simulink model "ee_motor_pmsm_drive"  (R2020b)
settings: Solver=ode23t  StartTime=0.0  StopTime=tsim  MaxStep=1e-6  RelTol=1e-4  AbsTol=1e-3  EnableMultiTasking=on
PreLoadFcn:
  | tsim = 0.05;
PostLoadFcn:
  | % Create the PMSM data
  | ee_motor_pmsm_drive_params
  | 
  | % Test harness test point
  | rpm0 = 1400;
  | torque0 = 200;
InitFcn:
  | % Set simulation time for 5 full AC cycles
  | tsim = 5*60/rpm0/N;
StopFcn:
  | ee_addSimlogTimeStamp(bdroot)
undefined symbols (not defined in the file): Imax, Ld, Lq, N, PM, Rs, Tmax, Ts, Tsc
libraries: ee_lib x22, fl_lib x12, nesl_utility x12, pid_lib x3, eeTransforms x2, eePwmGeneratorTwoLevel x1
(part 1 of 2)
CloseFcn:
  | try,close(h1_ee_motor_pmsm_drive),end
  | clear h1_ee_motor_pmsm_drive
  | try,close(h2_ee_motor_pmsm_drive),end
  | clear h2_ee_motor_pmsm_drive
  | try,close(h3_ee_motor_pmsm_drive),end
  | clear h3_ee_motor_pmsm_drive
  | try,close(h4_ee_motor_pmsm_drive),end
  | clear h4_ee_motor_pmsm_drive
  | 
  | 
  | clear simlog_ee_motor_pmsm_drive
  | clear logsout_ee_motor_pmsm_drive
  | clear Imax L0 Ld Lq N PM Pmax Rs Tmax TorqueMatrix Ts Tsc dfluxAdiaMatrix dfluxAdibMatrix dfluxAdicMatrix dfluxAdxMatrix efficiency fc fnom fsw iDC idVec iqVec omegam_nom powerDC powerLosses rpm0 rpm_nom t tMax tMin tabulatedLosses time torque0 totalLosses tout tsim vDC xVec
Description:
  | HEV PMSM Drive Test Harness
settings Model: Creator=The MathWorks, Inc.  LastModifiedBy=ge62gas
settings SolverCC: AutoScaleAbsTol=off  MaxConsecutiveMinStep=2
settings DataIOCC: LimitDataPoints=on  MaxDataPoints=35000  SaveFormat=StructureWithTime  SaveOutput=off  DSMLogging=off  ReturnWorkspaceOutputs=off  SignalLoggingName=logsout_ee_motor_pmsm_drive
settings OptimizationCC: LifeSpan=inf
settings DebuggingCC: UnderspecifiedInitializationDetection=Classic  MergeDetectMultiDrivingBlocksExec=none  AllowSymbolicDim=off  PregeneratedLibrarySubsystemCodeDiagnostic=none  SFUnexpectedBacktrackingDiag=warning  SFNoUnconditionalDefaultTransitionDiag=warning  SFExecutionAtInitializationDiag=none  ArithmeticOperatorsInVariantConditions=warning
settings HardwareCC: ProdBitPerPointer=32  ProdBitPerSizeT=32  ProdBitPerPtrDiffT=32  ProdLargestAtomicFloat=None  ProdIntDivRoundTo=Undefined  ProdEndianess=Unspecified  ProdWordSize=32  ProdHWDeviceType=32-bit Generic
settings ModelReferenceCC: PropagateSignalLabelsOutOfModel=off
settings SFSimCC: SimUseLocalCustomCode=off
settings RTWCC: RTWUseLocalCustomCode=off
settings CodeAppCC: StateflowObjectComments=on
settings GRTTargetCC: TargetLangStandard=C89/C90 (ANSI)
settings ConfigComp: CovMetricSettings=dw  CovSaveCumulativeToWorkspaceVar=on  CovSaveSingleToWorkspaceVar=on  CovExternalEMLEnable=off  CovSFcnEnable=off
settings SimscapeCC: SimscapeLogType=all  SimscapeLogSimulationStatistics=on  SimscapeLogName=simlog_ee_motor_pmsm_drive  SimscapeLogDecimation=10  SimscapeLogDataHistory=1000000

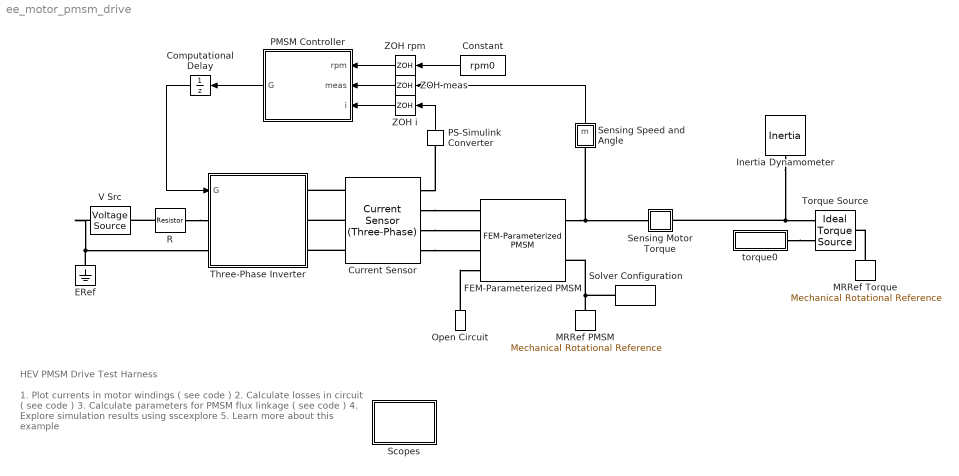
== system ee_motor_pmsm_drive ==
  note: HEV PMSM Drive Test Harness
  note: 1. Plot currents in motor windings ( see code )
      | 2. Calculate losses in circuit ( see code )
      | 3. Calculate parameters for PMSM flux linkage ( see code )
      | 4. Explore simulation results using sscexplore
      | 5. Learn more about this example
  Computational Delay : UnitDelay  SampleTime=Ts  HasFrameUpgradeWarning=on
  Constant : Constant  Value=rpm0
  Current Sensor : ee_lib/Sensors & Transducers/Current Sensor (Three-Phase)
      settings: SourceProductName=Electrical  InternalSimscapePortConfiguration="{\"Bottom\":[],\"Left\":[{\"id\":\"a1\",\"label\":\"a1\",\"type\":\"foundation.electrical.electrical\"},{\"id\":\"b1\",\"label\":\"b1\",\"type\":\"foundation.electrical.electrical\"},{\"id\":\"c1\",\"label\":\"c1\",\"type\":\"foundation.electrical.electrical\"}],\"Right\":[{\"id\":\"I_output\",\"label\":\"I\",\"type\":\"output\"},{\"id\":\"a2\",\"label\":\"a2\",\"type\":\"foundation.electrical.electrical\"},{\"id\":\"b2\",\"label\":\"b2\",\"type\":\"foundation.electrical.electrical\"},{\"id\":\"c2\",\"label\":\"c2\",\"type\":\"foundation.electrical.electrical\"}],\"Top\":[]}"
  ERef : fl_lib/Electrical/Electrical Elements/Electrical Reference
      settings: SourceProductName=Foundation Library
  FEM-Parameterized PMSM : ee_lib/Electromechanical/Permanent Magnet/FEM-Parameterized PMSM  parameterization=1  winding_type=ee.enum.statorconnection.wye  iVec=[-2, 0, 2] A  xVec=xVec rad  dfluxdiMatrix=0.0002 * ones(3, 4) Wb/A  dfluxdxMatrix=[0, -.16, .16, 0; 0, -.16, .16, 0; 0, -.16, .16, 0] Wb/rad  calculate_torque_matrix=1  TorqueMatrix=zeros(3, 3, 3, 4) N*m  idVec1=[-200, 0, 200] A  iqVec1=[-200, 0, 200] A  LdMatrix=0.0002 * ones(3, 3) H  LqMatrix=0.0002 * ones(3, 3) H  PmMatrix=0.1 * ones(3, 3) Wb  N=6  interp_method=simscape.enum.interpolation.smooth  Rs=Rs Ohm  Ms=0.00002 H  L0=0.00016 H  losses_oc=[500 1500 0] W  losses_sc=[200 600 0] W  f_losses=140 Hz  Isc_losses=350 A  Inertia=0.01 kg*m^2  lam=0 N*m/(rad/s)  i_d_specify=on  i_d_priority=High  i_d=0 A  i_d_nominal_specify=off  i_d_nominal_unit=A  i_d_nominal_value=1  i_q_specify=on  i_q_priority=High  i_q=0 A  i_q_nominal_specify=off  i_q_nominal_unit=A  i_q_nominal_value=1  torque_specify=off  torque_priority=None  torque=0 N*m  torque_nominal_specify=off  torque_nominal_unit=N*m  torque_nominal_value=1  angular_velocity_specify=on  angular_velocity_priority=High  angular_velocity=rpm0 rpm  angular_velocity_nominal_specify=off  angular_velocity_nominal_unit=rpm  angular_velocity_nominal_value=1  angular_position_specify=on  angular_position_priority=High  angular_position=-pi/2/N rad  angular_position_nominal_specify=off  angular_position_nominal_unit=deg  angular_position_nominal_value=1  Tmeas=298.15 K  alpha=3.93e-3 1/K  alpha_flux=-0.001 1/K  stator_thermal_mass=100 J/K  stator_initial_temperatures=[298.15, 298.15, 298.15] K  rotor_thermal_mass=200 J/K  rotor_initial_temperature=298.15 K  Rm_percent_rotor=90  Rd_percent_rotor=30  idVec=idVec A  iqVec=iqVec A  dfluxAdiaMatrix3D=dfluxAdiaMatrix Wb/A  dfluxAdibMatrix3D=dfluxAdibMatrix Wb/A  dfluxAdicMatrix3D=dfluxAdicMatrix Wb/A  dfluxAdxMatrix3D=dfluxAdxMatrix Wb/rad  TorqueMatrix3D=TorqueMatrix N*m  iaVec=[-200, 0, 200] A  ibVec=[-200, 0, 200] A  icVec=[-200, 0, 200] A  dfluxAdiaMatrix=zeros(3, 3, 3, 4) Wb/A  dfluxAdibMatrix=zeros(3, 3, 3, 4) Wb/A  dfluxAdicMatrix=zeros(3, 3, 3, 4) Wb/A  dfluxAdxMatrix=zeros(3, 3, 3, 4) Wb/rad  param_dq0=1  winding_type_dq0=1  nPolePairs=4  parks_type=1  idVec2=[-200, 0, 200] A  iqVec2=[-200, 0, 200] A  magVec2=[0, 100, 200] A  betaVec2=[-180, -90, 0, 90, 180] deg  xVec2=[0, 5, 10, 15, 20, 25, 30] deg  fluxD_dq0=zeros(3, 3, 7) Wb  fluxQ_dq0=zeros(3, 3, 7) Wb  fluxA_dq0=zeros(3, 3, 7) Wb  Torque_dq0=zeros(3, 3, 7) N*m  fluxD_IBX=zeros(3, 5, 7) Wb  fluxQ_IBX=zeros(3, 5, 7) Wb  fluxA_IBX=zeros(3, 5, 7) Wb  Torque_IBX=zeros(3, 5, 7) N*m
      settings: SourceProductName=Electrical  LogSimulationData=on  InternalSimscapePortConfiguration="{\"Bottom\":[],\"Left\":[{\"id\":\"a\",\"label\":\"a\",\"type\":\"foundation.electrical.electrical\"},{\"id\":\"b\",\"label\":\"b\",\"type\":\"foundation.electrical.electrical\"},{\"id\":\"c\",\"label\":\"c\",\"type\":\"foundation.electrical.electrical\"},{\"id\":\"n\",\"label\":\"n\",\"type\":\"foundation.electrical.electrical\"}],\"Right\":[{\"id\":\"R\",\"label\":\"R\",\"type\":\"foundation.mechanical.rotational.rotational\"},{\"id\":\"C\",\"label\":\"C\",\"type\":\"foundation.mechanical.rotational.rotational\"}],\"Top\":[]}"
  Inertia Dynamometer : fl_lib/Mechanical/Rotational Elements/Inertia  inertia=1 kg*m^2  num_ports=foundation.enum.numPorts2.one  w_specify=on  w_priority=High  w=rpm0 rpm  w_nominal_specify=off  w_nominal_unit=rad/s  w_nominal_value=1  t_specify=off  t_priority=High  t=0 N*m  t_nominal_specify=off  t_nominal_unit=N*m  t_nominal_value=1
      settings: SourceProductName=Foundation Library
  MRRef PMSM : fl_lib/Mechanical/Rotational Elements/Mechanical Rotational Reference
      settings: SourceProductName=Foundation Library
  MRRef Torque : fl_lib/Mechanical/Rotational Elements/Mechanical Rotational Reference
      settings: SourceProductName=Foundation Library
  Open Circuit : fl_lib/Electrical/Electrical Elements/Open Circuit  v_specify=off  v_priority=None  v=0 V  v_nominal_specify=off  v_nominal_unit=V  v_nominal_value=1
      settings: SourceProductName=Foundation Library
  PMSM Controller : Subsystem
  PS-Simulink Converter : nesl_utility/PS-Simulink Converter  PhysicalDomain=network_engine_domain  SubClassName=ps_output  LeftPortType=input  RightPortType=output  PseudoPeriodic=off  Frequencies=[]  Unit=A  AffineConversion=off
      settings: SourceProductName=Utilities
  R : fl_lib/Electrical/Electrical Elements/Resistor  R=0.01 Ohm  i_specify=off  i_priority=None  i=0 A  i_nominal_specify=off  i_nominal_unit=A  i_nominal_value=1  v_specify=off  v_priority=None  v=0 V  v_nominal_specify=off  v_nominal_unit=V  v_nominal_value=1
      settings: SourceProductName=Foundation Library
  Scopes : Subsystem
  Sensing Motor Torque : Subsystem
      mask Display: disp('trq');
  Sensing Speed and Angle : Subsystem
      mask Display: disp('m')
  Solver Configuration : nesl_utility/Solver Configuration  PhysicalDomain=network_engine_domain  SubClassName=solver  LeftPortType=input  RightPortType=generic  Tones=[]  Harmonics=[]  SimulateNoise=off  Profile=off  UseLocalSampling=off  EnableSwitchedLinearOptims=on  FrequencyDomain=off  UseCCode=off  RelTol=0.001  AbsTol=1e-06  MinStep=1e-09  ToWorkspace=off  RevertToSquareIcSolve=off  NumHomotopyIterations=100  PhasorMode=off  PhasorModeNumHarmonics=1  DoDC=off  ResidualTolerance=1e-9  UseLocalSolver=off  LocalSolverChoice=NE_BACKWARD_EULER_ADVANCER  LocalSolverSampleTime=Ts/1000  DoFixedCost=on  MaxNonlinIter=4  MaxModeIter=2  ComputeImpulses=off  ImpulseIterations=2  LinearAlgebra=auto  EquationFormulation=NE_TIME_EF  DelaysMemoryBudget=1024  AutomaticFiltering=on  FilteringTimeConstant=0.001  PartitionStorageMethod=AS_NEEDED  PartitionMemoryBudget=1024  PartitionMethod=FAST
      settings: SourceProductName=Utilities
  Three-Phase Inverter : Subsystem  Tag=PublishSubsystem
  Torque Source : fl_lib/Mechanical/Mechanical Sources/Ideal Torque Source
      settings: SourceProductName=Foundation Library
  V Src : ee_lib/Sources/Voltage Source  dc_voltage=500 V  ac_voltage=0 V  ac_shift=0 deg  ac_frequency=0 Hz  noise_mode=0  PSD=0 V^2/Hz  repeatability=1  auto_seed=529650792  user_seed=0  sample_time=0.001 s  i_specify=off  i_priority=None  i=0 A  i_nominal_specify=off  i_nominal_unit=A  i_nominal_value=1  v_specify=off  v_priority=None  v=0 V  v_nominal_specify=off  v_nominal_unit=V  v_nominal_value=1
      settings: AttributesFormatString=%<dc_voltage> %<dc_voltage_unit>  SourceProductName=Electrical
  ZOH i : ZeroOrderHold  SampleTime=Tsc
  ZOH meas : ZeroOrderHold  SampleTime=Tsc
  ZOH rpm : ZeroOrderHold  SampleTime=Tsc
  torque0 : Subsystem
      mask Display: disp('torque0');
  wires:
  PMSM Controller/1(G) -> Computational Delay/1
  ZOH i/1 -> PMSM Controller/3(i)
  Computational Delay/1 -> Three-Phase Inverter/1(G)
  ZOH meas/1 -> PMSM Controller/2(meas)
  ZOH rpm/1 -> PMSM Controller/1(rpm)
  Sensing Speed and Angle/1(m) -> ZOH meas/1
  Constant/1 -> ZOH rpm/1
  PS-Simulink Converter/1 -> ZOH i/1
  connections:
  FEM-Parameterized PMSM/RConn1 -- Sensing Speed and Angle/LConn1 -- Sensing Motor Torque/LConn1
  V Src/RConn1 -- Three-Phase Inverter/LConn2 -- ERef/LConn1
  Current Sensor/LConn1 -- Three-Phase Inverter/RConn1
  Current Sensor/RConn2 -- FEM-Parameterized PMSM/LConn1
  Current Sensor/LConn2 -- Three-Phase Inverter/RConn2
  Current Sensor/RConn3 -- FEM-Parameterized PMSM/LConn2
  Current Sensor/LConn3 -- Three-Phase Inverter/RConn3
  Current Sensor/RConn4 -- FEM-Parameterized PMSM/LConn3
  Inertia Dynamometer/LConn1 -- Sensing Motor Torque/RConn1 -- Torque Source/RConn2
  R/LConn1 -- V Src/LConn1
  R/RConn1 -- Three-Phase Inverter/LConn1
  MRRef PMSM/LConn1 -- Solver Configuration/RConn1 -- FEM-Parameterized PMSM/RConn2
  Open Circuit/LConn1 -- FEM-Parameterized PMSM/LConn4
  MRRef Torque/LConn1 -- Torque Source/LConn1
  torque0/RConn1 -- Torque Source/RConn1
  Current Sensor/RConn1 -- PS-Simulink Converter/LConn1

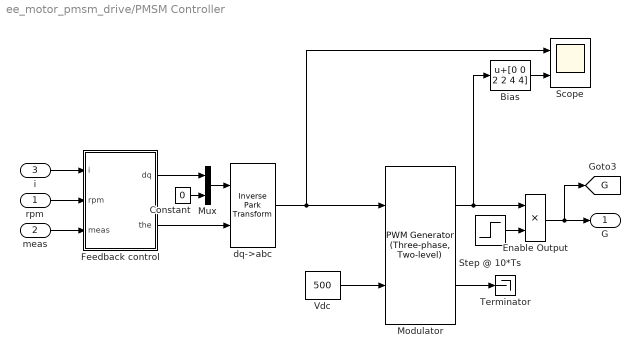
== system ee_motor_pmsm_drive/PMSM Controller ==
  rpm : Inport
  meas : Inport  Port=2
  i : Inport  Port=3
  Bias : Bias  Bias=[0 0 2 2 4 4]
  Constant : Constant  Value=0  SampleTime=-1
  Enable Output : Product
  Feedback control : Subsystem
  Modulator : eePwmGeneratorTwoLevel/PWM Generator (Three-phase, Two-level)  PWMMode=Continuous PWM (CPWM)  CPWMMode=SPWM: sinusoidal PWM  DPWMMode=60 DPWM: 60 degree discontinuous PWM  fsw=fsw  Ts=Ts
      settings: SourceProductBaseCode=PS
  Mux : Mux  Inputs=2
  Scope : Scope  NumInputPorts=2
  Step @ 10*Ts : Step  Time=10*Ts  SampleTime=Ts
  Terminator : Terminator
  Vdc : Constant  Value=500  SampleTime=Tsc
  dq->abc : eeTransforms/Inverse Park Transform  AxisAlignment=Q-axis  PowerInvariant=off
  G : Outport  VectorParamsAs1DForOutWhenUnconnected=off
  tag scope: G=global
  wires:
  dq->abc/1 -> Scope/1, Modulator/1
  Vdc/1 -> Modulator/2
  Step @ 10*Ts/1 -> Enable Output/2
  Modulator/2 -> Terminator/1
  i/1 -> Feedback control/1(i)
  rpm/1 -> Feedback control/2(rpm)
  meas/1 -> Feedback control/3(meas)
  Feedback control/2(the) -> dq->abc/2
  Modulator/1 -> Bias/1, Enable Output/1
  Enable Output/1 -> [G], G/1
  Constant/1 -> Mux/2
  Mux/1 -> dq->abc/1
  Feedback control/1(dq) -> Mux/1
  Bias/1 -> Scope/2

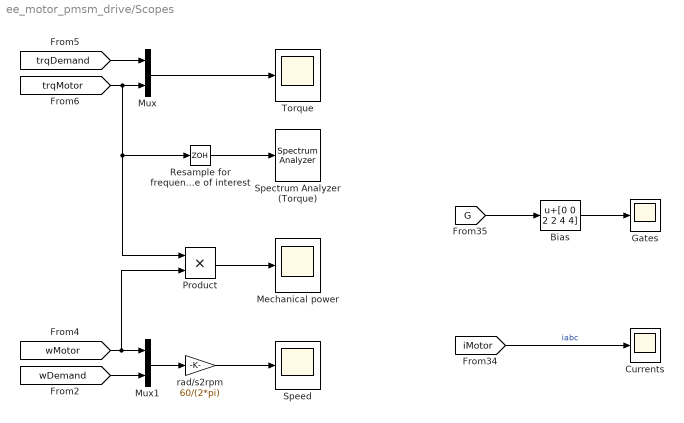
== system ee_motor_pmsm_drive/Scopes ==
  Bias : Bias  Bias=[0 0 2 2 4 4]
  Currents : Scope
  Gates : Scope
  Mechanical power : Scope
  Mux : Mux  Inputs=2
  Mux1 : Mux  Inputs=2
  Product : Product
  Resample for frequency range of interest : ZeroOrderHold  SampleTime=2.5e-5
  Spectrum Analyzer (Torque) : SpectrumAnalyzer  Tag=PublishScope
  Speed : Scope
  Torque : Scope
  rad/s2rpm : Gain  Gain=60/(2*pi)
  wires:
  rad/s2rpm/1 -> Speed/1
  Mux/1 -> Torque/1
  [iMotor] -> Currents/1  "iabc"
  [trqDemand] -> Mux/1
  Mux1/1 -> rad/s2rpm/1
  [wMotor] -> Mux1/1, Product/2
  [G] -> Bias/1
  Bias/1 -> Gates/1
  Product/1 -> Mechanical power/1
  Resample for frequency range of interest/1 -> Spectrum Analyzer (Torque)/1
  [wDemand] -> Mux1/2
  [trqMotor] -> Product/1, Resample for frequency range of interest/1, Mux/2

== system ee_motor_pmsm_drive/Sensing Motor Torque ==
  Ideal Torque Sensor : fl_lib/Mechanical/Mechanical Sensors/Ideal Torque Sensor
      settings: SourceProductName=Foundation Library
  PS-Simulink Converter2 : nesl_utility/PS-Simulink Converter  PhysicalDomain=network_engine_domain  SubClassName=ps_output  LeftPortType=input  RightPortType=output  PseudoPeriodic=off  Frequencies=[]  Unit=N*m  AffineConversion=off
      settings: SourceProductName=Utilities
  R : PMIOPort  Side=Left
  C : PMIOPort  Port=2  Side=Right
  tag scope: trqMotor=global
  wires:
  PS-Simulink Converter2/1 -> [trqMotor]
  connections:
  Ideal Torque Sensor/RConn2 -- PS-Simulink Converter2/LConn1
  R/RConn1 -- Ideal Torque Sensor/LConn1
  Ideal Torque Sensor/RConn1 -- C/RConn1

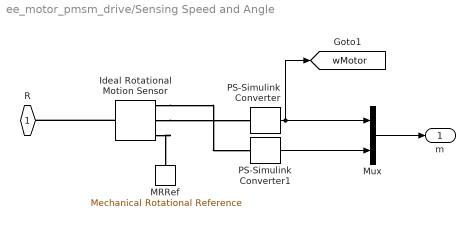
== system ee_motor_pmsm_drive/Sensing Speed and Angle ==
  Ideal Rotational Motion Sensor : fl_lib/Mechanical/Mechanical Sensors/Ideal Rotational Motion Sensor  wrap_angle=simscape.enum.onoff.off  offset=0 deg
      settings: SourceProductName=Foundation Library
  MRRef : fl_lib/Mechanical/Rotational Elements/Mechanical Rotational Reference
      settings: SourceProductName=Foundation Library
  Mux : Mux  Inputs=2
  PS-Simulink Converter : nesl_utility/PS-Simulink Converter  PhysicalDomain=network_engine_domain  SubClassName=ps_output  LeftPortType=input  RightPortType=output  PseudoPeriodic=off  Frequencies=[]  Unit=rad/s  AffineConversion=off
      settings: SourceProductName=Utilities
  PS-Simulink Converter1 : nesl_utility/PS-Simulink Converter  PhysicalDomain=network_engine_domain  SubClassName=ps_output  LeftPortType=input  RightPortType=output  PseudoPeriodic=off  Frequencies=[]  Unit=rad  AffineConversion=off
      settings: SourceProductName=Utilities
  R : PMIOPort  Side=Left
  m : Outport  VectorParamsAs1DForOutWhenUnconnected=off
  tag scope: wMotor=global
  wires:
  Mux/1 -> m/1
  PS-Simulink Converter/1 -> Mux/1, [wMotor]
  PS-Simulink Converter1/1 -> Mux/2
  connections:
  Ideal Rotational Motion Sensor/RConn3 -- PS-Simulink Converter1/LConn1
  Ideal Rotational Motion Sensor/RConn1 -- MRRef/LConn1
  Ideal Rotational Motion Sensor/RConn2 -- PS-Simulink Converter/LConn1
  Ideal Rotational Motion Sensor/LConn1 -- R/RConn1

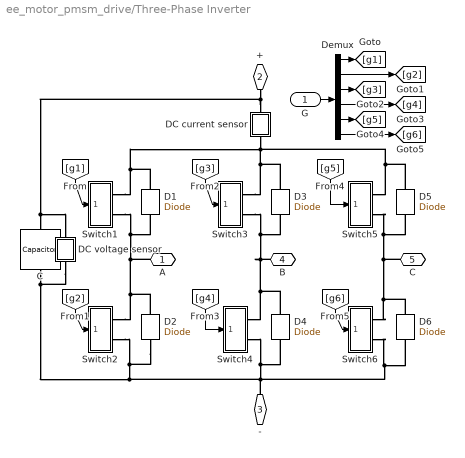
== system ee_motor_pmsm_drive/Three-Phase Inverter ==
  G : Inport
  " C" : ee_lib/Passive/Capacitor  cap_option=0  c=10 F  Cvec=[ 1e-5 1e-6 ] F  Vvec=[ 0 10 ] V  CV_table_symmetry=1  f_vec=[1, 10] kHz  DFext_vec=[.8, 1.2]  C_tol=5  enable_C_tol=0  tol_distribution=1  nSigma=4  r=0.001 Ohm  g=0 1/Ohm  averaging_period=0 s  enable_operating_limits=0  operating_limit_action=2  max_working_voltage_range=[ -25 25 ] V  power_rating=1 W  enable_faults=0  fault_action=1  Cscale_faulted=100  R_faulted=0.001 Ohm  G_faulted=0 1/Ohm  tau_fault=0.001 s  enable_temporal_fault=0  t_fault=1 s  enable_behavioral_fault=0  max_permissible_voltage_range=[ -100 100 ] V  t_fail_on_voltage=1 s  i_specify=off  i_priority=Low  i=0 A  i_nominal_specify=off  i_nominal_unit=A  i_nominal_value=1  v_specify=off  v_priority=None  v=0 V  v_nominal_specify=off  v_nominal_unit=V  v_nominal_value=1  vc_specify=on  vc_priority=High  vc=500 V  vc_nominal_specify=off  vc_nominal_unit=V  vc_nominal_value=1
      settings: SourceProductName=Electrical
  D{1..6} (6 alike) : ee_lib/Semiconductors & Converters/Diode  ModelType=ee.enum.diode.modelType.exponential  IfMat=[.07, .12, .19, 1.75, 4.24, 7.32, 11.2; .16, .3, .72, 2.14, 4.02, 6.35, 9.12] A  TjVec=[25, 125] degC  VfVec=[.5, .7, .9, 1.3, 1.7, 2.1, 2.5] V  Vf=0.6 V  Ron=0.3 Ohm  Goff=1e-8 S  prmExp=2  I12=[ 0.0137 0.545 ] A  V12=[ 0.6 0.7 ] V  IS=1e-7 A  ec=1  I1=0.0137 A  V1=0.6 V  RS=0.001 Ohm  Tmeas=25 degC  N_series=1  N_parallel=1  Rz=0.3 Ohm  BV=Inf V  C_param=1  CJ=50 pF  CJ0=50 pF  VJ=1 V  Mgrad=0.5  Vvec=[ 0.1 10 100 ] V  Cvec=[ 3.5 1 0.4 ] pF  FC=0.5  Q_param=ee.enum.diode.recoveryParam.off  iRM=-7.15 A  iF=4 A  didt=-750 A/us  trr_factor=3  trr=115 ns  Qrr=1500 s*uA  TT=50 ns  tau=100 ns  T_param=1  IS_T2=1.25e-7 A  I1_T2=0.245 A  V1_T2=0.5 V  Tmeas2=125 degC  EG_param=1  EG=1.11 eV  XTI_param=1  XTI=3  dBVdT=0 V/K  Tdevice=25 degC  i_specify=off  i_priority=None  i=0 A  i_nominal_specify=off  i_nominal_unit=A  i_nominal_value=1  v_specify=off  v_priority=None  v=0 V  v_nominal_specify=off  v_nominal_unit=V  v_nominal_value=1  i_capacitor_specify=off  i_capacitor_priority=High  i_capacitor=0 A  i_capacitor_nominal_specify=off  i_capacitor_nominal_unit=A  i_capacitor_nominal_value=1  v_capacitor_specify=off  v_capacitor_priority=None  v_capacitor=0 V  v_capacitor_nominal_specify=off  v_capacitor_nominal_unit=V  v_capacitor_nominal_value=1  power_dissipated_specify=off  power_dissipated_priority=None  power_dissipated=0 W  power_dissipated_nominal_specify=off  power_dissipated_nominal_unit=W  power_dissipated_nominal_value=1  thermal_network_parameterization=ee.enum.thermalNetworkTopology.cauer  Rth=[0, 10] K/W  Rth_Foster=[4, 6] K/W  thermal_mass_parameterization=ee.enum.thermalNetwork.timeconstant  thermal_mass=[0, 1] J/K  thermal_mass_Foster=[1.5, 3] J/K  thermal_time_constant=[0, 10] s  thermal_time_constant_Foster=[6, 18] s  thermal_mass_initial_temperatures=[25, 25] degC
      settings: SourceProductName=Electrical  LogSimulationData=on
  DC current sensor : Subsystem
      mask Display: disp('i');
  DC voltage sensor : Subsystem
      mask Display: disp('v')
  Demux : Demux  Outputs=6
  Switch1 : Subsystem
  Switch2 : Subsystem
  Switch3 : Subsystem
  Switch4 : Subsystem
  Switch5 : Subsystem
  Switch6 : Subsystem
  A : PMIOPort  Tag=PMCPort  Side=Right
  + : PMIOPort  Tag=PMCPort  Port=2  Side=Left
  - : PMIOPort  Tag=PMCPort  Port=3  Side=Left
  B : PMIOPort  Tag=PMCPort  Port=4  Side=Right
  C : PMIOPort  Tag=PMCPort  Port=5  Side=Right
  wires:
  Demux/6 -> [g6]
  Demux/5 -> [g5]
  Demux/4 -> [g4]
  Demux/3 -> [g3]
  Demux/2 -> [g2]
  G/1 -> Demux/1
  Demux/1 -> [g1]
  [g1] -> Switch1/1(g)
  [g2] -> Switch2/1(g)
  [g3] -> Switch3/1(g)
  [g4] -> Switch4/1(g)
  [g5] -> Switch5/1(g)
  [g6] -> Switch6/1(g)
  connections:
  -/RConn1 -- D6/LConn1 -- Switch6/RConn2 -- Switch4/RConn2 -- D4/LConn1 -- DC voltage sensor/LConn1 -- " C"/RConn1 -- D2/LConn1 -- Switch2/RConn2
  A/RConn1 -- Switch1/RConn2 -- D1/LConn1 -- D2/RConn1 -- Switch2/RConn1
  B/RConn1 -- Switch4/RConn1 -- D4/RConn1 -- Switch3/RConn2 -- D3/LConn1
  C/RConn1 -- Switch6/RConn1 -- D6/RConn1 -- Switch5/RConn2 -- D5/LConn1
  +/RConn1 -- DC voltage sensor/RConn1 -- " C"/LConn1 -- DC current sensor/RConn1
  D3/RConn1 -- Switch3/RConn1 -- Switch1/RConn1 -- D1/RConn1 -- DC current sensor/LConn1 -- Switch5/RConn1 -- D5/RConn1

== system ee_motor_pmsm_drive/torque0 ==
  Constant1 : Constant  Value=torque0
  Simulink-PS Converter : nesl_utility/Simulink-PS Converter  PhysicalDomain=network_engine_domain  SubClassName=ps_input  LeftPortType=input  RightPortType=output  PseudoPeriodic=off  Frequencies=[]  NoiseDistribution=none  NoiseParameters=[]  Unit=N*m  AffineConversion=off  FilteringAndDerivatives=zero  SimscapeFilterOrder=1  InputFilterTimeConstant=0.001  UdotUserProvided=1
      settings: SourceProductName=Utilities
  R : PMIOPort  Side=Right
  tag scope: trqDemand=global
  wires:
  Constant1/1 -> Simulink-PS Converter/1, [trqDemand]
  connections:
  Simulink-PS Converter/RConn1 -- R/RConn1

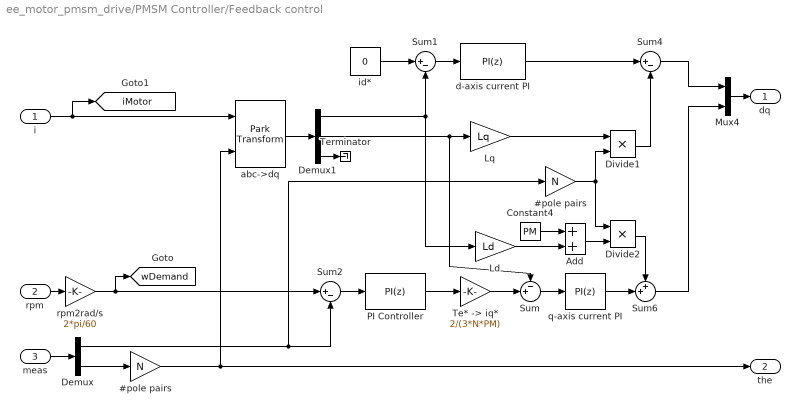
== system ee_motor_pmsm_drive/PMSM Controller/Feedback control ==
  i : Inport
  rpm : Inport  Port=2
  meas : Inport  Port=3
  " #pole pairs " : Gain  Gain=N
  #pole pairs : Gain  Gain=N
  Add : Sum
  Constant4 : Constant  Value=PM  SampleTime=Tsc
  Demux : Demux  Outputs=2
  Demux1 : Demux  Outputs=3
  Divide1 : Product  Inputs=**
  Divide2 : Product  Inputs=**
  Ld : Gain  Gain=Ld
  Lq : Gain  Gain=Lq
  Mux4 : Mux  Inputs=2
  PI Controller : pid_lib/PID Controller  Controller=PI  Form=Parallel  TimeDomain=Discrete-time  UseExternalTs=off  SampleTime=Tsc  IntegratorMethod=Forward Euler  FilterMethod=Forward Euler  ControllerParametersSource=internal  P=120  I=1200  D=0  UseFilter=on  N=100  TunerSelectOption=Transfer Function Based (PID Tuner App)  InitialConditionSource=internal  InitialConditionForIntegrator=torque0  InitialConditionForFilter=0  DifferentiatorICPrevScaledInput=0  ExternalReset=none  TrackingMode=off  Kt=1  LimitOutput=on  SatLimitsSource=internal  UpperSaturationLimit=Tmax*1.5  LowerSaturationLimit=-Tmax*1.5  LinearizeAsGain=on  AntiWindupMode=back-calculation  Kb=1000  POutMin=[]  POutMax=[]  IOutMin=[]  IOutMax=[]  DOutMin=[]  DOutMax=[]  NOutMin=[]  NOutMax=[]  SumOutMin=[]  SumOutMax=[]  SaturationOutMin=[]  SaturationOutMax=[]  PParamMin=[]  PParamMax=[]  IParamMin=[]  IParamMax=[]  DParamMin=[]  DParamMax=[]  NParamMin=[]  NParamMax=[]  KbParamMin=[]  KbParamMax=[]  KtParamMin=[]  KtParamMax=[]  KbOutMin=[]  KbOutMax=[]  KtOutMin=[]  KtOutMax=[]  IntegratorOutMin=[]  IntegratorOutMax=[]  FilterOutMin=[]  FilterOutMax=[]  SumI1OutMin=[]  SumI1OutMax=[]  SumI2OutMin=[]  SumI2OutMax=[]  SumI3OutMin=[]  SumI3OutMax=[]  SumI4OutMin=[]  SumI4OutMax=[]  SumDOutMin=[]  SumDOutMax=[]  DifferentiatorOutMin=[]  DifferentiatorOutMax=[]  FilterDiffOutCoefMin=[]  FilterDiffOutCoefMax=[]  ReciprocalOutMin=[]  ReciprocalOutMax=[]  SumDenOutMin=[]  SumDenOutMax=[]  SumNumOutMin=[]  SumNumOutMax=[]  DivideOutMin=[]  DivideOutMax=[]  UdiffTsProdOutMin=[]  UdiffTsProdOutMax=[]  NTsProdOutMin=[]  NTsProdOutMax=[]  UintegralTsProdOutMin=[]  UintegralTsProdOutMax=[]  UngainTsProdOutMin=[]  UngainTsProdOutMax=[]  IntegratorContinuousStateAttributes=''  IntegratorStateMustResolveToSignalObject=off  IntegratorRTWStateStorageClass=Auto  FilterContinuousStateAttributes=''  FilterStateMustResolveToSignalObject=off  FilterRTWStateStorageClass=Auto  ParallelPVariant=InternalParameters  IdealPVariant=Disabled  IVariant=InternalParameters  DVariant=Disabled  IntegratorVariant=Discrete  SatVariant=Enabled  AWVariant=BackCalculation  PCopyVariant=Disabled  TRVariant=Disabled  FdbkBlocksVariant=Forward  IdealPFdbkVariant=Disabled  SatFdbkVariant=Disabled  DerivativeFilterVariant=Disabled  NVariant=Disabled  NCopyVariant=Disabled_SignalSpec  FilterICVariant=Disabled  IntegratorICVariant=InternalICs  ExternalResetVariant=Disabled  TRSumVariant=Passthrough  SumFdbkVariant=Disabled  SumVariant=Sum_PI  TsampFilterVariant=InternalTs  TsampNgainVariant=Passthrough  TsampIntegralVariant=Passthrough  ExternalSaturationOutDataTypeStr=Inherit: Same as second input
  Sum : Sum  Inputs=-+|
  Sum1 : Sum  Inputs=|+-
  Sum2 : Sum  Inputs=|+-
  Sum4 : Sum  Inputs=|+-
  Sum6 : Sum  Inputs=++|
  "Te* -> iq*" : Gain  Gain=2/(3*N*PM)
  Terminator : Terminator
  abc->dq : eeTransforms/Park Transform  AxisAlignment=Q-axis  PowerInvariant=off
  d-axis current PI : pid_lib/PID Controller  Controller=PI  Form=Parallel  TimeDomain=Discrete-time  UseExternalTs=off  SampleTime=Tsc  IntegratorMethod=Forward Euler  FilterMethod=Forward Euler  ControllerParametersSource=internal  P=0.1  I=10  D=0  UseFilter=on  N=100  TunerSelectOption=Transfer Function Based (PID Tuner App)  InitialConditionSource=internal  InitialConditionForIntegrator=0  InitialConditionForFilter=0  DifferentiatorICPrevScaledInput=0  ExternalReset=none  TrackingMode=off  Kt=1  LimitOutput=on  SatLimitsSource=internal  UpperSaturationLimit=5*Rs*Imax  LowerSaturationLimit=-5*Rs*Imax  LinearizeAsGain=on  AntiWindupMode=back-calculation  Kb=1000  POutMin=[]  POutMax=[]  IOutMin=[]  IOutMax=[]  DOutMin=[]  DOutMax=[]  NOutMin=[]  NOutMax=[]  SumOutMin=[]  SumOutMax=[]  SaturationOutMin=[]  SaturationOutMax=[]  PParamMin=[]  PParamMax=[]  IParamMin=[]  IParamMax=[]  DParamMin=[]  DParamMax=[]  NParamMin=[]  NParamMax=[]  KbParamMin=[]  KbParamMax=[]  KtParamMin=[]  KtParamMax=[]  KbOutMin=[]  KbOutMax=[]  KtOutMin=[]  KtOutMax=[]  IntegratorOutMin=[]  IntegratorOutMax=[]  FilterOutMin=[]  FilterOutMax=[]  SumI1OutMin=[]  SumI1OutMax=[]  SumI2OutMin=[]  SumI2OutMax=[]  SumI3OutMin=[]  SumI3OutMax=[]  SumI4OutMin=[]  SumI4OutMax=[]  SumDOutMin=[]  SumDOutMax=[]  DifferentiatorOutMin=[]  DifferentiatorOutMax=[]  FilterDiffOutCoefMin=[]  FilterDiffOutCoefMax=[]  ReciprocalOutMin=[]  ReciprocalOutMax=[]  SumDenOutMin=[]  SumDenOutMax=[]  SumNumOutMin=[]  SumNumOutMax=[]  DivideOutMin=[]  DivideOutMax=[]  UdiffTsProdOutMin=[]  UdiffTsProdOutMax=[]  NTsProdOutMin=[]  NTsProdOutMax=[]  UintegralTsProdOutMin=[]  UintegralTsProdOutMax=[]  UngainTsProdOutMin=[]  UngainTsProdOutMax=[]  IntegratorContinuousStateAttributes=''  IntegratorStateMustResolveToSignalObject=off  IntegratorRTWStateStorageClass=Auto  FilterContinuousStateAttributes=''  FilterStateMustResolveToSignalObject=off  FilterRTWStateStorageClass=Auto  ParallelPVariant=InternalParameters  IdealPVariant=Disabled  IVariant=InternalParameters  DVariant=Disabled  IntegratorVariant=Discrete  SatVariant=Enabled  AWVariant=BackCalculation  PCopyVariant=Disabled  TRVariant=Disabled  FdbkBlocksVariant=Forward  IdealPFdbkVariant=Disabled  SatFdbkVariant=Disabled  DerivativeFilterVariant=Disabled  NVariant=Disabled  NCopyVariant=Disabled_SignalSpec  FilterICVariant=Disabled  IntegratorICVariant=InternalICs  ExternalResetVariant=Disabled  TRSumVariant=Passthrough  SumFdbkVariant=Disabled  SumVariant=Sum_PI  TsampFilterVariant=InternalTs  TsampNgainVariant=Passthrough  TsampIntegralVariant=Passthrough  ExternalSaturationOutDataTypeStr=Inherit: Same as second input
  id* : Constant  Value=0  SampleTime=Tsc
  q-axis current PI : pid_lib/PID Controller  Controller=PI  Form=Parallel  TimeDomain=Discrete-time  UseExternalTs=off  SampleTime=Tsc  IntegratorMethod=Forward Euler  FilterMethod=Forward Euler  ControllerParametersSource=internal  P=0.1  I=10  D=0.000539029417831173  UseFilter=on  N=29631.0341187165  TunerSelectOption=Transfer Function Based (PID Tuner App)  InitialConditionSource=internal  InitialConditionForIntegrator=0  InitialConditionForFilter=0  DifferentiatorICPrevScaledInput=0  ExternalReset=none  TrackingMode=off  Kt=1  LimitOutput=on  SatLimitsSource=internal  UpperSaturationLimit=5*Rs*Imax  LowerSaturationLimit=-5*Rs*Imax  LinearizeAsGain=on  AntiWindupMode=back-calculation  Kb=1000  POutMin=[]  POutMax=[]  IOutMin=[]  IOutMax=[]  DOutMin=[]  DOutMax=[]  NOutMin=[]  NOutMax=[]  SumOutMin=[]  SumOutMax=[]  SaturationOutMin=[]  SaturationOutMax=[]  PParamMin=[]  PParamMax=[]  IParamMin=[]  IParamMax=[]  DParamMin=[]  DParamMax=[]  NParamMin=[]  NParamMax=[]  KbParamMin=[]  KbParamMax=[]  KtParamMin=[]  KtParamMax=[]  KbOutMin=[]  KbOutMax=[]  KtOutMin=[]  KtOutMax=[]  IntegratorOutMin=[]  IntegratorOutMax=[]  FilterOutMin=[]  FilterOutMax=[]  SumI1OutMin=[]  SumI1OutMax=[]  SumI2OutMin=[]  SumI2OutMax=[]  SumI3OutMin=[]  SumI3OutMax=[]  SumI4OutMin=[]  SumI4OutMax=[]  SumDOutMin=[]  SumDOutMax=[]  DifferentiatorOutMin=[]  DifferentiatorOutMax=[]  FilterDiffOutCoefMin=[]  FilterDiffOutCoefMax=[]  ReciprocalOutMin=[]  ReciprocalOutMax=[]  SumDenOutMin=[]  SumDenOutMax=[]  SumNumOutMin=[]  SumNumOutMax=[]  DivideOutMin=[]  DivideOutMax=[]  UdiffTsProdOutMin=[]  UdiffTsProdOutMax=[]  NTsProdOutMin=[]  NTsProdOutMax=[]  UintegralTsProdOutMin=[]  UintegralTsProdOutMax=[]  UngainTsProdOutMin=[]  UngainTsProdOutMax=[]  IntegratorContinuousStateAttributes=''  IntegratorStateMustResolveToSignalObject=off  IntegratorRTWStateStorageClass=Auto  FilterContinuousStateAttributes=''  FilterStateMustResolveToSignalObject=off  FilterRTWStateStorageClass=Auto  ParallelPVariant=InternalParameters  IdealPVariant=Disabled  IVariant=InternalParameters  DVariant=Disabled  IntegratorVariant=Discrete  SatVariant=Enabled  AWVariant=BackCalculation  PCopyVariant=Disabled  TRVariant=Disabled  FdbkBlocksVariant=Forward  IdealPFdbkVariant=Disabled  SatFdbkVariant=Disabled  DerivativeFilterVariant=Disabled  NVariant=Disabled  NCopyVariant=Disabled_SignalSpec  FilterICVariant=Disabled  IntegratorICVariant=InternalICs  ExternalResetVariant=Disabled  TRSumVariant=Passthrough  SumFdbkVariant=Disabled  SumVariant=Sum_PI  TsampFilterVariant=InternalTs  TsampNgainVariant=Passthrough  TsampIntegralVariant=Passthrough  ExternalSaturationOutDataTypeStr=Inherit: Same as second input
  rpm2rad/s : Gain  Gain=2*pi/60
  dq : Outport  VectorParamsAs1DForOutWhenUnconnected=off
  the : Outport  Port=2  VectorParamsAs1DForOutWhenUnconnected=off
  tag scope: iMotor=global, wDemand=global
  wires:
  abc->dq/1 -> Demux1/1
  Sum4/1 -> Mux4/1
  Demux/2 -> " #pole pairs "/1
  i/1 -> abc->dq/1, [iMotor]
  PI Controller/1 -> "Te* -> iq*"/1
  Constant4/1 -> Add/1
  Add/1 -> Divide2/2
  Demux1/1 -> Ld/1, Sum1/2
  meas/1 -> Demux/1
  rpm/1 -> rpm2rad/s/1
  d-axis current PI/1 -> Sum4/1
  Sum2/1 -> PI Controller/1
  Sum1/1 -> d-axis current PI/1
  Sum6/1 -> Mux4/2
  id*/1 -> Sum1/1
  Ld/1 -> Add/2
  #pole pairs/1 -> Divide2/1, Divide1/2
  Sum/1 -> q-axis current PI/1
  "Te* -> iq*"/1 -> Sum/2
  Divide2/1 -> Sum6/1
  " #pole pairs "/1 -> the/1, abc->dq/2
  q-axis current PI/1 -> Sum6/2
  Demux1/2 -> Sum/1, Lq/1
  rpm2rad/s/1 -> Sum2/1, [wDemand]
  Demux/1 -> Sum2/2, #pole pairs/1
  Mux4/1 -> dq/1
  Lq/1 -> Divide1/1
  Divide1/1 -> Sum4/2
  Demux1/3 -> Terminator/1

== system ee_motor_pmsm_drive/Three-Phase Inverter/DC current sensor ==
  Current Sensor : fl_lib/Electrical/Electrical Sensors/Current Sensor
      settings: SourceProductName=Foundation Library  LogSimulationData=on
  - : PMIOPort  Side=Left
  + : PMIOPort  Port=2  Side=Right
  connections:
  +/RConn1 -- Current Sensor/LConn1
  Current Sensor/RConn2 -- -/RConn1

== system ee_motor_pmsm_drive/Three-Phase Inverter/DC voltage sensor ==
  Voltage Sensor : fl_lib/Electrical/Electrical Sensors/Voltage Sensor
      settings: SourceProductName=Foundation Library  LogSimulationData=on
  - : PMIOPort  Side=Left
  + : PMIOPort  Port=2  Side=Right
  connections:
  Voltage Sensor/RConn2 -- -/RConn1
  Voltage Sensor/LConn1 -- +/RConn1

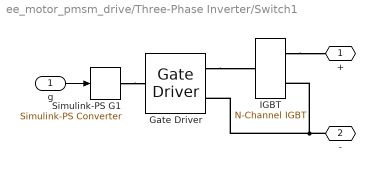
== system ee_motor_pmsm_drive/Three-Phase Inverter/Switch1 ==
  g : Inport
  Gate Driver : ee_lib/Semiconductors & Converters/Gate Driver  vHigh=15 V  vLow=0 V  parameterization=1  rHigh=10 Ohm  rLow=1 Ohm  tRise=20 ns  tFall=20 ns  cLoad=10 nF  enable_faults=0  t_fault=1 s  fault_type=1  uHighValue=0.7  uLowValue=0.3  tHigh=4 us  tLow=0 us  ZonTime_specify=off  ZonTime_priority=None  ZonTime=0 s  ZoffTime_specify=off  ZoffTime_priority=None  ZoffTime=0 s  uHigh=2.0 V  uLow=0.8 V
      settings: SourceProductName=Electrical  InternalSimscapePortConfiguration="{\"Bottom\":[],\"Left\":[{\"id\":\"u\",\"label\":\"u\",\"type\":\"input\"}],\"Right\":[{\"id\":\"G\",\"label\":\"G\",\"type\":\"foundation.electrical.electrical\"},{\"id\":\"S\",\"label\":\"S\",\"type\":\"foundation.electrical.electrical\"}],\"Top\":[]}"
  IGBT : ee_lib/Semiconductors & Converters/N-Channel IGBT  model_type=2  Ices=2 mA  Vces=600 V  Vth=6 V  Vce_sat=2.6 V  Ice_sat=400 A  Vge_sat=10 V  ec=1  Tmeas=25 degC  Vge_vec=[ -2 6 7 8 10 12 15 20 ] V  Vce_vec=[ -1 0 0.5 1 1.5 2 2.5 3 3.5 4 ] V  T_vec=[25, 125] degC  Ic_mat=[ -1.015e-5 1.35e-8 4.7135e-4 5.092e-4 5.105e-4 5.117500000000001e-4 5.1299e-4 5.1423e-4 5.1548e-4 5.1672e-4; -9.986899999999999e-6 1.35e-8 4.7135e-4 5.092e-4 5.105e-4 5.117500000000001e-4 5.1299e-4 5.1423e-4 5.1548e-4 5.1672e-4; -9.955e-6 1.35e-8 0.0065225 3.3324 48.154 93.661 105.52 105.72 105.93 106.14; -9.955e-6 1.35e-8 0.0065235 3.5783 70.264 166.33 252.4 317.67 353.38 357.39; -9.955e-6 1.35e-8 0.006524 3.7206 89.17100000000001 228.09 371.63 511.02 642.6900000000001 764.04; -9.9549e-6 1.35e-8 0.0065242 3.7716 97.79300000000001 256.21 424.27 592.92 759.2 921.52; -9.9549e-6 1.35e-8 0.0065243 3.8067 104.52 278.11 464.6 654.37 844.5700000000001 1.0339e+3; -9.9549e-6 1.35e-8 0.0065244 3.8324 109.92 295.67 496.54 702.28 909.96 1.1183e+3 ] A  Ic_mat_3D=zeros(8, 10, 2) A  C_param=1  C_GE=23.7 nF  C_GC=2.7 nF  C_CE=0 nF  C_ies=26.4 nF  C_res=2.7 nF  C_oes=0 nF  C_GE_vec=[ 25 31 26.5 24.9 25 24.9 24.6 24.7 24.8 ] nF  C_GC_vec=[ 55 9 5.5 3.1 2.5 2.1 1.9 1.8 1.7 ] nF  C_CE_vec=[ 5 11 6.5 4.9 3.5 2.7 2.1 1.7 1.4 ] nF  C_ies_vec=[ 80 40 32 28 27.5 27 26.5 26.5 26.5 ] nF  C_res_vec=[ 55 9 5.5 3.1 2.5 2.1 1.9 1.8 1.7 ] nF  C_oes_vec=[ 60 20 12 8 6 4.8 4 3.5 3.1 ] nF  C_Vce_vec=[ 0 1 2 5 10 15 20 25 30 ] V  charge_linearity_param=1  C_OX=20 nF  V_C_OX=-5 V  TF=0 us  VAF=200 V  RC=0.001 Ohm  RE=0.001 Ohm  RG=0.001 Ohm  BF=50  T_param=1  Ices_T2=100 mA  EG=1.11 eV  Vce_sat_T2=3 V  Tmeas2=125 degC  XTI=3  BEX=-1.5  RG_alpha=0 1/K  Tdevice=25 degC  Tdevice_3D=25 degC  thermal_network_parameterization=ee.enum.thermalNetworkTopology.cauer  Rth=[0, 10] K/W  Rth_Foster=[4, 6] K/W  thermal_mass_parameterization=1  thermal_mass=[0, 1] J/K  thermal_mass_Foster=[1.5, 3] J/K  thermal_time_constant=[0, 10] s  thermal_time_constant_Foster=[6, 18] s  thermal_mass_initial_temperatures=[298.15, 298.15] K  Ic_vec1=[0, 10, 50, 100, 200, 400, 600] A  Vce_vec1=[0, 1.1, 1.3, 1.45, 1.75, 2.25, 2.7] V  Rmiller=0.1 Ohm  Goff=1e-5 1/Ohm  t_on=0.07 us  t_rise=0.7 us  t_off=0.2 us  t_fall=0.5 us  v_meas=300 V  Tj_vec1=[298.15, 398.15] K  Vce_mat1=[0, 1.1, 1.3, 1.45, 1.75, 2.25, 2.7; 0, 1, 1.15, 1.35, 1.7, 2.35, 3] V  E_turn_on_mat1=[0, .2, 1, 2, 4, 8, 15; 0, .3, 1.3, 2.5, 5, 11, 18] * 1e-3 J  E_turn_off_mat1=[0, .3, 1.5, 3, 6, 15, 25; 0, .7, 3.3, 6.5, 13, 25, 35] * 1e-3 J
      settings: SourceProductName=Electrical  LogSimulationData=on  InternalSimscapePortConfiguration="{\"Bottom\":[],\"Left\":[{\"id\":\"G\",\"label\":\"\",\"type\":\"foundation.electrical.electrical\"}],\"Right\":[{\"id\":\"C\",\"label\":\"\",\"type\":\"foundation.electrical.electrical\"},{\"id\":\"E\",\"label\":\"\",\"type\":\"foundation.electrical.electrical\"}],\"Top\":[]}"
  Simulink-PS G1 : nesl_utility/Simulink-PS Converter  PhysicalDomain=network_engine_domain  SubClassName=ps_input  LeftPortType=input  RightPortType=output  PseudoPeriodic=off  Frequencies=[]  NoiseDistribution=none  NoiseParameters=[]  Unit=1  AffineConversion=off  FilteringAndDerivatives=zero  SimscapeFilterOrder=1  InputFilterTimeConstant=1e-6  UdotUserProvided=0
      settings: SourceProductName=Utilities
  + : PMIOPort  Side=Right
  - : PMIOPort  Port=2  Side=Right
  wires:
  g/1 -> Simulink-PS G1/1
  connections:
  IGBT/RConn1 -- +/RConn1
  -/RConn1 -- IGBT/RConn2 -- Gate Driver/RConn2
  Gate Driver/RConn1 -- IGBT/LConn1
  Simulink-PS G1/RConn1 -- Gate Driver/LConn1

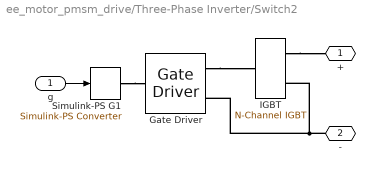
== system ee_motor_pmsm_drive/Three-Phase Inverter/Switch2 ==
  g : Inport
  Gate Driver : ee_lib/Semiconductors & Converters/Gate Driver  vHigh=15 V  vLow=0 V  parameterization=1  rHigh=10 Ohm  rLow=1 Ohm  tRise=20 ns  tFall=20 ns  cLoad=10 nF  enable_faults=0  t_fault=1 s  fault_type=1  uHighValue=0.7  uLowValue=0.3  tHigh=4 us  tLow=0 us  ZonTime_specify=off  ZonTime_priority=None  ZonTime=0 s  ZoffTime_specify=off  ZoffTime_priority=None  ZoffTime=0 s  uHigh=2.0 V  uLow=0.8 V
      settings: SourceProductName=Electrical  InternalSimscapePortConfiguration="{\"Bottom\":[],\"Left\":[{\"id\":\"u\",\"label\":\"u\",\"type\":\"input\"}],\"Right\":[{\"id\":\"G\",\"label\":\"G\",\"type\":\"foundation.electrical.electrical\"},{\"id\":\"S\",\"label\":\"S\",\"type\":\"foundation.electrical.electrical\"}],\"Top\":[]}"
  IGBT : ee_lib/Semiconductors & Converters/N-Channel IGBT  model_type=2  Ices=2 mA  Vces=600 V  Vth=6 V  Vce_sat=2.6 V  Ice_sat=400 A  Vge_sat=10 V  ec=1  Tmeas=25 degC  Vge_vec=[ -2 6 7 8 10 12 15 20 ] V  Vce_vec=[ -1 0 0.5 1 1.5 2 2.5 3 3.5 4 ] V  T_vec=[25, 125] degC  Ic_mat=[ -1.015e-5 1.35e-8 4.7135e-4 5.092e-4 5.105e-4 5.117500000000001e-4 5.1299e-4 5.1423e-4 5.1548e-4 5.1672e-4; -9.986899999999999e-6 1.35e-8 4.7135e-4 5.092e-4 5.105e-4 5.117500000000001e-4 5.1299e-4 5.1423e-4 5.1548e-4 5.1672e-4; -9.955e-6 1.35e-8 0.0065225 3.3324 48.154 93.661 105.52 105.72 105.93 106.14; -9.955e-6 1.35e-8 0.0065235 3.5783 70.264 166.33 252.4 317.67 353.38 357.39; -9.955e-6 1.35e-8 0.006524 3.7206 89.17100000000001 228.09 371.63 511.02 642.6900000000001 764.04; -9.9549e-6 1.35e-8 0.0065242 3.7716 97.79300000000001 256.21 424.27 592.92 759.2 921.52; -9.9549e-6 1.35e-8 0.0065243 3.8067 104.52 278.11 464.6 654.37 844.5700000000001 1.0339e+3; -9.9549e-6 1.35e-8 0.0065244 3.8324 109.92 295.67 496.54 702.28 909.96 1.1183e+3 ] A  Ic_mat_3D=zeros(8, 10, 2) A  C_param=1  C_GE=23.7 nF  C_GC=2.7 nF  C_CE=0 nF  C_ies=26.4 nF  C_res=2.7 nF  C_oes=0 nF  C_GE_vec=[ 25 31 26.5 24.9 25 24.9 24.6 24.7 24.8 ] nF  C_GC_vec=[ 55 9 5.5 3.1 2.5 2.1 1.9 1.8 1.7 ] nF  C_CE_vec=[ 5 11 6.5 4.9 3.5 2.7 2.1 1.7 1.4 ] nF  C_ies_vec=[ 80 40 32 28 27.5 27 26.5 26.5 26.5 ] nF  C_res_vec=[ 55 9 5.5 3.1 2.5 2.1 1.9 1.8 1.7 ] nF  C_oes_vec=[ 60 20 12 8 6 4.8 4 3.5 3.1 ] nF  C_Vce_vec=[ 0 1 2 5 10 15 20 25 30 ] V  charge_linearity_param=1  C_OX=20 nF  V_C_OX=-5 V  TF=0 us  VAF=200 V  RC=0.001 Ohm  RE=0.001 Ohm  RG=0.001 Ohm  BF=50  T_param=1  Ices_T2=100 mA  EG=1.11 eV  Vce_sat_T2=3 V  Tmeas2=125 degC  XTI=3  BEX=-1.5  RG_alpha=0 1/K  Tdevice=25 degC  Tdevice_3D=25 degC  thermal_network_parameterization=ee.enum.thermalNetworkTopology.cauer  Rth=[0, 10] K/W  Rth_Foster=[4, 6] K/W  thermal_mass_parameterization=1  thermal_mass=[0, 1] J/K  thermal_mass_Foster=[1.5, 3] J/K  thermal_time_constant=[0, 10] s  thermal_time_constant_Foster=[6, 18] s  thermal_mass_initial_temperatures=[298.15, 298.15] K  Ic_vec1=[0, 10, 50, 100, 200, 400, 600] A  Vce_vec1=[0, 1.1, 1.3, 1.45, 1.75, 2.25, 2.7] V  Rmiller=0.1 Ohm  Goff=1e-5 1/Ohm  t_on=0.07 us  t_rise=0.7 us  t_off=0.2 us  t_fall=0.5 us  v_meas=300 V  Tj_vec1=[298.15, 398.15] K  Vce_mat1=[0, 1.1, 1.3, 1.45, 1.75, 2.25, 2.7; 0, 1, 1.15, 1.35, 1.7, 2.35, 3] V  E_turn_on_mat1=[0, .2, 1, 2, 4, 8, 15; 0, .3, 1.3, 2.5, 5, 11, 18] * 1e-3 J  E_turn_off_mat1=[0, .3, 1.5, 3, 6, 15, 25; 0, .7, 3.3, 6.5, 13, 25, 35] * 1e-3 J
      settings: SourceProductName=Electrical  LogSimulationData=on  InternalSimscapePortConfiguration="{\"Bottom\":[],\"Left\":[{\"id\":\"G\",\"label\":\"\",\"type\":\"foundation.electrical.electrical\"}],\"Right\":[{\"id\":\"C\",\"label\":\"\",\"type\":\"foundation.electrical.electrical\"},{\"id\":\"E\",\"label\":\"\",\"type\":\"foundation.electrical.electrical\"}],\"Top\":[]}"
  Simulink-PS G1 : nesl_utility/Simulink-PS Converter  PhysicalDomain=network_engine_domain  SubClassName=ps_input  LeftPortType=input  RightPortType=output  PseudoPeriodic=off  Frequencies=[]  NoiseDistribution=none  NoiseParameters=[]  Unit=1  AffineConversion=off  FilteringAndDerivatives=zero  SimscapeFilterOrder=1  InputFilterTimeConstant=1e-6  UdotUserProvided=0
      settings: SourceProductName=Utilities
  + : PMIOPort  Side=Right
  - : PMIOPort  Port=2  Side=Right
  wires:
  g/1 -> Simulink-PS G1/1
  connections:
  Simulink-PS G1/RConn1 -- Gate Driver/LConn1
  Gate Driver/RConn1 -- IGBT/LConn1
  IGBT/RConn2 -- -/RConn1 -- Gate Driver/RConn2
  IGBT/RConn1 -- +/RConn1

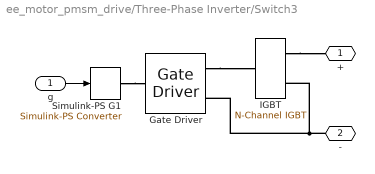
== system ee_motor_pmsm_drive/Three-Phase Inverter/Switch3 ==
  g : Inport
  Gate Driver : ee_lib/Semiconductors & Converters/Gate Driver  vHigh=15 V  vLow=0 V  parameterization=1  rHigh=10 Ohm  rLow=1 Ohm  tRise=20 ns  tFall=20 ns  cLoad=10 nF  enable_faults=0  t_fault=1 s  fault_type=1  uHighValue=0.7  uLowValue=0.3  tHigh=4 us  tLow=0 us  ZonTime_specify=off  ZonTime_priority=None  ZonTime=0 s  ZoffTime_specify=off  ZoffTime_priority=None  ZoffTime=0 s  uHigh=2.0 V  uLow=0.8 V
      settings: SourceProductName=Electrical  InternalSimscapePortConfiguration="{\"Bottom\":[],\"Left\":[{\"id\":\"u\",\"label\":\"u\",\"type\":\"input\"}],\"Right\":[{\"id\":\"G\",\"label\":\"G\",\"type\":\"foundation.electrical.electrical\"},{\"id\":\"S\",\"label\":\"S\",\"type\":\"foundation.electrical.electrical\"}],\"Top\":[]}"
  IGBT : ee_lib/Semiconductors & Converters/N-Channel IGBT  model_type=2  Ices=2 mA  Vces=600 V  Vth=6 V  Vce_sat=2.6 V  Ice_sat=400 A  Vge_sat=10 V  ec=1  Tmeas=25 degC  Vge_vec=[ -2 6 7 8 10 12 15 20 ] V  Vce_vec=[ -1 0 0.5 1 1.5 2 2.5 3 3.5 4 ] V  T_vec=[25, 125] degC  Ic_mat=[ -1.015e-5 1.35e-8 4.7135e-4 5.092e-4 5.105e-4 5.117500000000001e-4 5.1299e-4 5.1423e-4 5.1548e-4 5.1672e-4; -9.986899999999999e-6 1.35e-8 4.7135e-4 5.092e-4 5.105e-4 5.117500000000001e-4 5.1299e-4 5.1423e-4 5.1548e-4 5.1672e-4; -9.955e-6 1.35e-8 0.0065225 3.3324 48.154 93.661 105.52 105.72 105.93 106.14; -9.955e-6 1.35e-8 0.0065235 3.5783 70.264 166.33 252.4 317.67 353.38 357.39; -9.955e-6 1.35e-8 0.006524 3.7206 89.17100000000001 228.09 371.63 511.02 642.6900000000001 764.04; -9.9549e-6 1.35e-8 0.0065242 3.7716 97.79300000000001 256.21 424.27 592.92 759.2 921.52; -9.9549e-6 1.35e-8 0.0065243 3.8067 104.52 278.11 464.6 654.37 844.5700000000001 1.0339e+3; -9.9549e-6 1.35e-8 0.0065244 3.8324 109.92 295.67 496.54 702.28 909.96 1.1183e+3 ] A  Ic_mat_3D=zeros(8, 10, 2) A  C_param=1  C_GE=23.7 nF  C_GC=2.7 nF  C_CE=0 nF  C_ies=26.4 nF  C_res=2.7 nF  C_oes=0 nF  C_GE_vec=[ 25 31 26.5 24.9 25 24.9 24.6 24.7 24.8 ] nF  C_GC_vec=[ 55 9 5.5 3.1 2.5 2.1 1.9 1.8 1.7 ] nF  C_CE_vec=[ 5 11 6.5 4.9 3.5 2.7 2.1 1.7 1.4 ] nF  C_ies_vec=[ 80 40 32 28 27.5 27 26.5 26.5 26.5 ] nF  C_res_vec=[ 55 9 5.5 3.1 2.5 2.1 1.9 1.8 1.7 ] nF  C_oes_vec=[ 60 20 12 8 6 4.8 4 3.5 3.1 ] nF  C_Vce_vec=[ 0 1 2 5 10 15 20 25 30 ] V  charge_linearity_param=1  C_OX=20 nF  V_C_OX=-5 V  TF=0 us  VAF=200 V  RC=0.001 Ohm  RE=0.001 Ohm  RG=0.001 Ohm  BF=50  T_param=1  Ices_T2=100 mA  EG=1.11 eV  Vce_sat_T2=3 V  Tmeas2=125 degC  XTI=3  BEX=-1.5  RG_alpha=0 1/K  Tdevice=25 degC  Tdevice_3D=25 degC  thermal_network_parameterization=ee.enum.thermalNetworkTopology.cauer  Rth=[0, 10] K/W  Rth_Foster=[4, 6] K/W  thermal_mass_parameterization=1  thermal_mass=[0, 1] J/K  thermal_mass_Foster=[1.5, 3] J/K  thermal_time_constant=[0, 10] s  thermal_time_constant_Foster=[6, 18] s  thermal_mass_initial_temperatures=[298.15, 298.15] K  Ic_vec1=[0, 10, 50, 100, 200, 400, 600] A  Vce_vec1=[0, 1.1, 1.3, 1.45, 1.75, 2.25, 2.7] V  Rmiller=0.1 Ohm  Goff=1e-5 1/Ohm  t_on=0.07 us  t_rise=0.7 us  t_off=0.2 us  t_fall=0.5 us  v_meas=300 V  Tj_vec1=[298.15, 398.15] K  Vce_mat1=[0, 1.1, 1.3, 1.45, 1.75, 2.25, 2.7; 0, 1, 1.15, 1.35, 1.7, 2.35, 3] V  E_turn_on_mat1=[0, .2, 1, 2, 4, 8, 15; 0, .3, 1.3, 2.5, 5, 11, 18] * 1e-3 J  E_turn_off_mat1=[0, .3, 1.5, 3, 6, 15, 25; 0, .7, 3.3, 6.5, 13, 25, 35] * 1e-3 J
      settings: SourceProductName=Electrical  LogSimulationData=on  InternalSimscapePortConfiguration="{\"Bottom\":[],\"Left\":[{\"id\":\"G\",\"label\":\"\",\"type\":\"foundation.electrical.electrical\"}],\"Right\":[{\"id\":\"C\",\"label\":\"\",\"type\":\"foundation.electrical.electrical\"},{\"id\":\"E\",\"label\":\"\",\"type\":\"foundation.electrical.electrical\"}],\"Top\":[]}"
  Simulink-PS G1 : nesl_utility/Simulink-PS Converter  PhysicalDomain=network_engine_domain  SubClassName=ps_input  LeftPortType=input  RightPortType=output  PseudoPeriodic=off  Frequencies=[]  NoiseDistribution=none  NoiseParameters=[]  Unit=1  AffineConversion=off  FilteringAndDerivatives=zero  SimscapeFilterOrder=1  InputFilterTimeConstant=1e-6  UdotUserProvided=0
      settings: SourceProductName=Utilities
  + : PMIOPort  Side=Right
  - : PMIOPort  Port=2  Side=Right
  wires:
  g/1 -> Simulink-PS G1/1
  connections:
  Simulink-PS G1/RConn1 -- Gate Driver/LConn1
  Gate Driver/RConn1 -- IGBT/LConn1
  IGBT/RConn2 -- -/RConn1 -- Gate Driver/RConn2
  IGBT/RConn1 -- +/RConn1

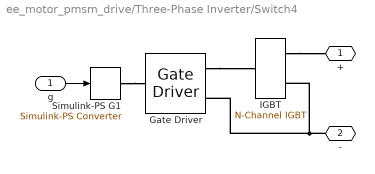
== system ee_motor_pmsm_drive/Three-Phase Inverter/Switch4 ==
  g : Inport
  Gate Driver : ee_lib/Semiconductors & Converters/Gate Driver  vHigh=15 V  vLow=0 V  parameterization=1  rHigh=10 Ohm  rLow=1 Ohm  tRise=20 ns  tFall=20 ns  cLoad=10 nF  enable_faults=0  t_fault=1 s  fault_type=1  uHighValue=0.7  uLowValue=0.3  tHigh=4 us  tLow=0 us  ZonTime_specify=off  ZonTime_priority=None  ZonTime=0 s  ZoffTime_specify=off  ZoffTime_priority=None  ZoffTime=0 s  uHigh=2.0 V  uLow=0.8 V
      settings: SourceProductName=Electrical  InternalSimscapePortConfiguration="{\"Bottom\":[],\"Left\":[{\"id\":\"u\",\"label\":\"u\",\"type\":\"input\"}],\"Right\":[{\"id\":\"G\",\"label\":\"G\",\"type\":\"foundation.electrical.electrical\"},{\"id\":\"S\",\"label\":\"S\",\"type\":\"foundation.electrical.electrical\"}],\"Top\":[]}"
  IGBT : ee_lib/Semiconductors & Converters/N-Channel IGBT  model_type=2  Ices=2 mA  Vces=600 V  Vth=6 V  Vce_sat=2.6 V  Ice_sat=400 A  Vge_sat=10 V  ec=1  Tmeas=25 degC  Vge_vec=[ -2 6 7 8 10 12 15 20 ] V  Vce_vec=[ -1 0 0.5 1 1.5 2 2.5 3 3.5 4 ] V  T_vec=[25, 125] degC  Ic_mat=[ -1.015e-5 1.35e-8 4.7135e-4 5.092e-4 5.105e-4 5.117500000000001e-4 5.1299e-4 5.1423e-4 5.1548e-4 5.1672e-4; -9.986899999999999e-6 1.35e-8 4.7135e-4 5.092e-4 5.105e-4 5.117500000000001e-4 5.1299e-4 5.1423e-4 5.1548e-4 5.1672e-4; -9.955e-6 1.35e-8 0.0065225 3.3324 48.154 93.661 105.52 105.72 105.93 106.14; -9.955e-6 1.35e-8 0.0065235 3.5783 70.264 166.33 252.4 317.67 353.38 357.39; -9.955e-6 1.35e-8 0.006524 3.7206 89.17100000000001 228.09 371.63 511.02 642.6900000000001 764.04; -9.9549e-6 1.35e-8 0.0065242 3.7716 97.79300000000001 256.21 424.27 592.92 759.2 921.52; -9.9549e-6 1.35e-8 0.0065243 3.8067 104.52 278.11 464.6 654.37 844.5700000000001 1.0339e+3; -9.9549e-6 1.35e-8 0.0065244 3.8324 109.92 295.67 496.54 702.28 909.96 1.1183e+3 ] A  Ic_mat_3D=zeros(8, 10, 2) A  C_param=1  C_GE=23.7 nF  C_GC=2.7 nF  C_CE=0 nF  C_ies=26.4 nF  C_res=2.7 nF  C_oes=0 nF  C_GE_vec=[ 25 31 26.5 24.9 25 24.9 24.6 24.7 24.8 ] nF  C_GC_vec=[ 55 9 5.5 3.1 2.5 2.1 1.9 1.8 1.7 ] nF  C_CE_vec=[ 5 11 6.5 4.9 3.5 2.7 2.1 1.7 1.4 ] nF  C_ies_vec=[ 80 40 32 28 27.5 27 26.5 26.5 26.5 ] nF  C_res_vec=[ 55 9 5.5 3.1 2.5 2.1 1.9 1.8 1.7 ] nF  C_oes_vec=[ 60 20 12 8 6 4.8 4 3.5 3.1 ] nF  C_Vce_vec=[ 0 1 2 5 10 15 20 25 30 ] V  charge_linearity_param=1  C_OX=20 nF  V_C_OX=-5 V  TF=0 us  VAF=200 V  RC=0.001 Ohm  RE=0.001 Ohm  RG=0.001 Ohm  BF=50  T_param=1  Ices_T2=100 mA  EG=1.11 eV  Vce_sat_T2=3 V  Tmeas2=125 degC  XTI=3  BEX=-1.5  RG_alpha=0 1/K  Tdevice=25 degC  Tdevice_3D=25 degC  thermal_network_parameterization=ee.enum.thermalNetworkTopology.cauer  Rth=[0, 10] K/W  Rth_Foster=[4, 6] K/W  thermal_mass_parameterization=1  thermal_mass=[0, 1] J/K  thermal_mass_Foster=[1.5, 3] J/K  thermal_time_constant=[0, 10] s  thermal_time_constant_Foster=[6, 18] s  thermal_mass_initial_temperatures=[298.15, 298.15] K  Ic_vec1=[0, 10, 50, 100, 200, 400, 600] A  Vce_vec1=[0, 1.1, 1.3, 1.45, 1.75, 2.25, 2.7] V  Rmiller=0.1 Ohm  Goff=1e-5 1/Ohm  t_on=0.07 us  t_rise=0.7 us  t_off=0.2 us  t_fall=0.5 us  v_meas=300 V  Tj_vec1=[298.15, 398.15] K  Vce_mat1=[0, 1.1, 1.3, 1.45, 1.75, 2.25, 2.7; 0, 1, 1.15, 1.35, 1.7, 2.35, 3] V  E_turn_on_mat1=[0, .2, 1, 2, 4, 8, 15; 0, .3, 1.3, 2.5, 5, 11, 18] * 1e-3 J  E_turn_off_mat1=[0, .3, 1.5, 3, 6, 15, 25; 0, .7, 3.3, 6.5, 13, 25, 35] * 1e-3 J
      settings: SourceProductName=Electrical  LogSimulationData=on  InternalSimscapePortConfiguration="{\"Bottom\":[],\"Left\":[{\"id\":\"G\",\"label\":\"\",\"type\":\"foundation.electrical.electrical\"}],\"Right\":[{\"id\":\"C\",\"label\":\"\",\"type\":\"foundation.electrical.electrical\"},{\"id\":\"E\",\"label\":\"\",\"type\":\"foundation.electrical.electrical\"}],\"Top\":[]}"
  Simulink-PS G1 : nesl_utility/Simulink-PS Converter  PhysicalDomain=network_engine_domain  SubClassName=ps_input  LeftPortType=input  RightPortType=output  PseudoPeriodic=off  Frequencies=[]  NoiseDistribution=none  NoiseParameters=[]  Unit=1  AffineConversion=off  FilteringAndDerivatives=zero  SimscapeFilterOrder=1  InputFilterTimeConstant=1e-6  UdotUserProvided=0
      settings: SourceProductName=Utilities
  + : PMIOPort  Side=Right
  - : PMIOPort  Port=2  Side=Right
  wires:
  g/1 -> Simulink-PS G1/1
  connections:
  IGBT/RConn1 -- +/RConn1
  Gate Driver/RConn2 -- -/RConn1 -- IGBT/RConn2
  Gate Driver/RConn1 -- IGBT/LConn1
  Simulink-PS G1/RConn1 -- Gate Driver/LConn1
